simulink model "re_mid_thust_test"  (R2024b)
settings: Solver=VariableStepAuto  StartTime=0.0  StopTime=50.0  RelTol=1e-3
InitFcn:
  | [moter_left, moter_right, moter_bow, A ,mass, boat_dimensions, friction, inertia] = get_parameters()
  | [K, B, thuster_angle] = re_LQR()
values from neighbouring files (symbols this model uses):
  friction = [-2, -1, -2]    [mid.m]
undefined symbols (not defined in the file or in its folder): inertia, mass, moter_bow, moter_left, moter_right
settings Model: Creator=klyx  LastModifiedBy=klyx

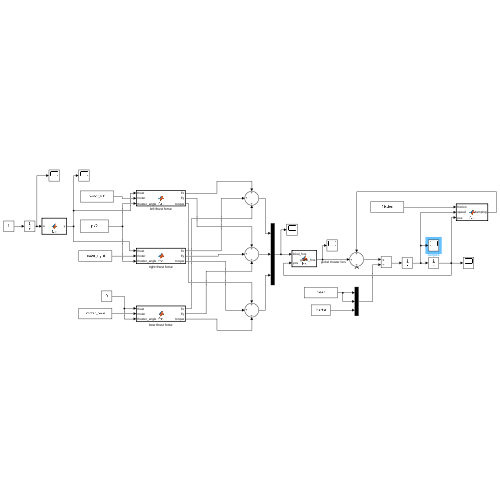
[thumbnail: Simulink's stored preview of the top-level diagram]
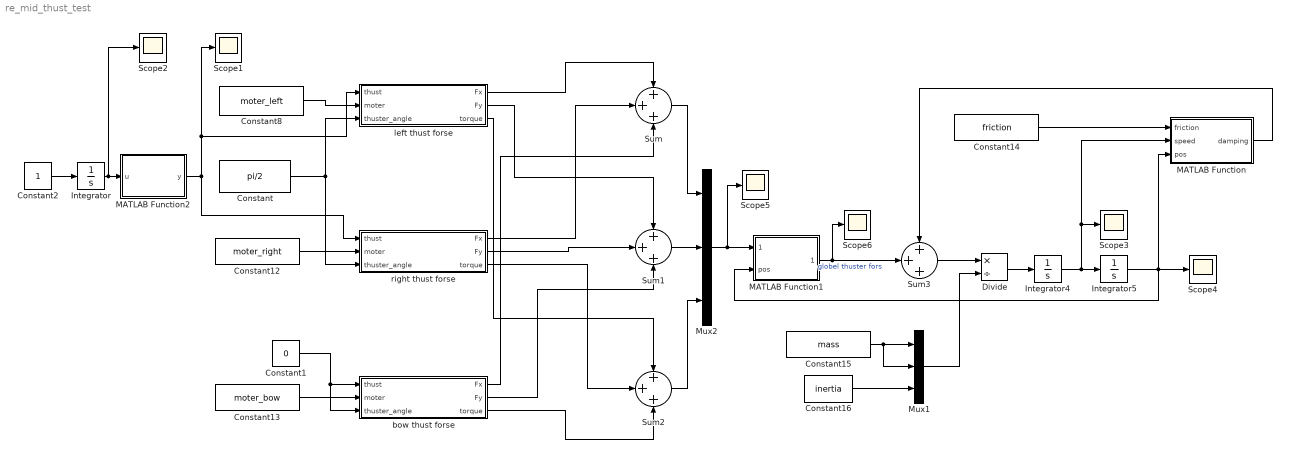
== system re_mid_thust_test ==
  Constant : Constant  Value=pi/2
  Constant1 : Constant  Value=0
  Constant12 : Constant  Value=moter_right
  Constant13 : Constant  Value=moter_bow
  Constant14 : Constant  Value=friction
  Constant15 : Constant  Value=mass
  Constant16 : Constant  Value=inertia
  Constant2 : Constant
  Constant8 : Constant  Value=moter_left
  Divide : Product  Inputs=*/
  Integrator : Integrator
  Integrator4 : Integrator  InitialCondition=[0; 0; 0]
  Integrator5 : Integrator  InitialCondition=[0; 0; pi/4]
  MATLAB Function : MATLAB Function  TreatAsAtomicUnit=on
  MATLAB Function1 : MATLAB Function  TreatAsAtomicUnit=on
  MATLAB Function2 : MATLAB Function  TreatAsAtomicUnit=on
  Mux1 : Mux  Inputs=3
  Mux2 : Mux  Inputs=3
  Scope{1..6} (6 alike) : Scope
  Sum{,1..3} (4 alike) : Sum  Inputs=+++
  bow thust forse : MATLAB Function  TreatAsAtomicUnit=on
  left thust forse : MATLAB Function  TreatAsAtomicUnit=on
  right thust forse : MATLAB Function  TreatAsAtomicUnit=on
  wires:
  right thust forse/2(Fy) -> Sum1/2
  Constant12/1 -> right thust forse/2(moter)
  bow thust forse/2(Fy) -> Sum1/3
  left thust forse/3(torque) -> Sum2/1
  Mux2/1 -> MATLAB Function1/1(lokal_fors), Scope5/1
  left thust forse/1(Fx) -> Sum/1
  right thust forse/1(Fx) -> Sum/2
  Integrator5/1 -> Scope4/1, MATLAB Function/3(pos), MATLAB Function1/2(pos)
  Constant13/1 -> bow thust forse/2(moter)
  left thust forse/2(Fy) -> Sum1/1
  right thust forse/3(torque) -> Sum2/2
  Constant8/1 -> left thust forse/2(moter)
  MATLAB Function1/1(globel_fors) -> Scope6/1, Sum3/2  "globel thuster fors"
  bow thust forse/3(torque) -> Sum2/3
  bow thust forse/1(Fx) -> Sum/3
  Sum/1 -> Mux2/1
  Sum1/1 -> Mux2/2
  Sum2/1 -> Mux2/3
  Sum3/1 -> Divide/1
  Constant15/1 -> Mux1/2, Mux1/1
  Mux1/1 -> Divide/2
  Constant16/1 -> Mux1/3
  MATLAB Function/1(damping) -> Sum3/1
  Constant14/1 -> MATLAB Function/1(friction)
  Divide/1 -> Integrator4/1
  Integrator4/1 -> Integrator5/1, Scope3/1, MATLAB Function/2(speed)
  Constant/1 -> right thust forse/3(thuster_angle), left thust forse/3(thuster_angle)
  Constant1/1 -> bow thust forse/3(thuster_angle), bow thust forse/1(thust)
  Constant2/1 -> Integrator/1
  Integrator/1 -> Scope2/1, MATLAB Function2/1(u)
  MATLAB Function2/1(y) -> right thust forse/1(thust), Scope1/1, left thust forse/1(thust)

== matlab function re_mid_thust_test/left thust forse ==
  data: thust input; Fx output; moter input; thuster_angle input; Fy output; torque output
function [Fx, Fy, torque]  = fcn(thust, moter, thuster_angle)
%this is the in the boat local frame
Fx     = cos(thuster_angle)*thust;
Fy     = sin(thuster_angle)*thust;
torque = sin(moter(3)+thuster_angle)*moter(4);
%fors_lokal = [Fx, Fy, torque];

== matlab function re_mid_thust_test/MATLAB Function ==
  data: friction input; damping output; speed input; pos input
function damping = fcn(friction, speed, pos)

firk = [friction(1) 0           0           ;
        0           friction(2) 0           ;
        0           0           friction(3)]

glo_to_lok = [cos(-pos(3)) -sin(-pos(3)) 0 ;
              sin(-pos(3)) cos(-pos(3))  0 ;
              0           0              1]

s = speed
rotl = inv(glo_to_lok)*firk*glo_to_lok;
damping = inv(glo_to_lok)*firk*glo_to_lok*speed;

== matlab function re_mid_thust_test/bow thust forse ==
  data: thust input; Fx output; moter input; thuster_angle input; Fy output; torque output
function [Fx, Fy, torque]  = fcn(thust, moter, thuster_angle)
%this is the in the boat local frame
Fx     = cos(thuster_angle)*thust;
Fy     = sin(thuster_angle)*thust;
torque = sin(moter(3)+thuster_angle)*moter(4);
%fors_lokal = [Fx, Fy, torque];

== matlab function re_mid_thust_test/right thust forse ==
  data: thust input; Fx output; moter input; thuster_angle input; Fy output; torque output
function [Fx, Fy, torque]  = fcn(thust, moter, thuster_angle)
%this is the in the boat local frame
Fx     = cos(thuster_angle)*thust;
Fy     = sin(thuster_angle)*thust;
torque = sin(moter(3)+thuster_angle)*moter(4);
%fors_lokal = [Fx, Fy, torque];

== matlab function re_mid_thust_test/MATLAB Function1 ==
  data: lokal_fors input; globel_fors output; pos input
function globel_fors = fcn(lokal_fors ,pos)

xy_pos = [lokal_fors(1);lokal_fors(2)];

glo_to_lok = [cos(pos(3)) -sin(pos(3));
              sin(pos(3)) cos(pos(3))];

gb_xy_fors = glo_to_lok*xy_pos;

globel_fors  = [gb_xy_fors(1);gb_xy_fors(2); 0];

== matlab function re_mid_thust_test/MATLAB Function2 ==
  data: u input; y output
function y = fcn(u)
if(u > 2)
    y = 0;
else
    y = 10;
end
